simulink model "MicroMouseMatlab"  (R2024b)
settings: Solver=FixedStepAuto  StartTime=0.0  StopTime=0.1  RelTol=1e-3  EnableMultiTasking=on
undefined symbols (not defined in the file): samplingTime
settings Model: STM32="{\"DigitalPortWrite\":[{\"ID\":\"MicroMouseTemplate:84:3\"},{\"ID\":\"MicroMouseTemplate:84:4\"},{\"ID\":\"MicroMouseTemplate:84:5\"},{\"ID\":\"MicroMouseTemplate:84:6\"},{\"ID\":\"MicroMouseTemplate:84:7\"},{\"ID\":\"MicroMouseTemplate:84:8\"},{\"ID\":\"MicroMouseTemplate:84:9\"},{\"ID\":\"MicroMouseTemplate:84:10\"},{\"ID\":\"MicroMouseTemplate:160:19\"},{\"ID\":\"MicroMouseTemplate:2479:4\"},{\"ID\":\"MicroMouseTemplate:2479:6\"},{\"ID\":\"MicroMouseTemplate:2479:7\"},{\"ID\":\"MicroMouseTemplate:2479:8\"}],\"PWMOutput\":[{\"ID\":\"MicroMouseTemplate:160:24\"},{\"ID\":\"MicroMouseTemplate:160:25\"}],\"AnalogInput\":{\"ID\":\"MicroMouseTemplate:2357:1\"},\"DigitalPortRead\":[{\"ID\":\"MicroMouseTemplate:2483:3\"},{\"ID\":\"MicroMouseTemplate:2483:4\"}]}"  SimulationMode=external  ExtModeTrigDuration=10  Creator=JesseJabezArendse
settings SolverCC: AllowMultiTaskInputOutput=on  AutoInsertRateTranBlk=on  InsertRTBMode=Never (minimum delay)
settings OptimizationCC: EnhancedBackFolding=on  PassReuseOutputArgsAs=Individual arguments  StateBitsets=on  DataBitsets=on  ZeroExternalMemoryAtStartup=off  ZeroInternalMemoryAtStartup=off  NoFixptDivByZeroProtection=on  MaxStackSize=512  OptimizeBlockOrder=speed  DifferentSizesBufferReuse=on  EfficientTunableParamExpr=on
settings DebuggingCC: MultiTaskCondExecSysMsg=none  ParameterOverflowMsg=none  ParameterPrecisionLossMsg=none  ParameterTunabilityLossMsg=error
settings HardwareCC: ProdBitPerPointer=32  ProdBitPerSizeT=32  ProdBitPerPtrDiffT=32  ProdLargestAtomicInteger=Long  ProdLargestAtomicFloat=Double  ProdWordSize=32  ProdLongLongMode=on  ProdHWDeviceType=ARM Compatible->ARM Cortex  TargetBitPerLong=64  TargetBitPerPointer=64  TargetBitPerSizeT=64  TargetBitPerPtrDiffT=64  TargetLongLongMode=on  TargetIntDivRoundTo=Zero  TargetEndianess=LittleEndian  TargetWordSize=64  TargetHWDeviceType=MATLAB Host
settings ModelReferenceCC: EnableParallelModelReferenceBuilds=on  ParallelModelReferenceMATLABWorkerInit=Copy Base Workspace  SupportModelReferenceSimTargetCustomCode=on
settings SFSimCC: MATLABDynamicMemAlloc=off  SimHardwareAcceleration=native
settings RTWCC: Description=Embedded Coder  SystemTargetFile=ert.tlc  HardwareBoard=STM32L4xx Based  TLCOptions=-p0 -aInlineSetEventsForThisBaseRateFcn=TLC_FALSE -aSuppressMultiTaskScheduler=TLC_FALSE -aRateBasedStepFcn=1  TemplateMakefile=ert_default_tmf  Toolchain=GNU Tools for ARM Embedded Processors  CodeExecutionProfiling=on  CodeProfilingInstrumentation=coarse  GPUComputeCapability=3.5
settings RTWCC: CustomHeaderCode=|
  | #include "MicroMouseProgramming\Core\Inc\IMU.h"
  | #include "MicroMouseProgramming\Core\Inc\CustomWhile.h"
  | #include "MicroMouseProgramming\Core\Inc\Motors.h"
settings RTWCC: CustomInclude=|
  | MicroMouseProgramming\Core\Inc\
  | MicroMouseProgramming\Core\Src\
settings RTWCC: CustomSource=|
  | MicroMouseProgramming\Core\Src\IMU.c
  | MicroMouseProgramming\Core\Src\CustomWhile.c
  | MicroMouseProgramming\Core\Src\Motors.c
settings CodeAppCC: ForceParamTrailComments=on  IgnoreCustomStorageClasses=off  OperatorAnnotations=on  SimulinkDataObjDesc=on  SFDataObjDesc=on  InsertBlockDesc=on
settings ERTTargetCC: CodeReplacementLibrary=ARM Cortex-M  SupportNonFinite=off  SupportComplex=off  ExtModeTransport=3  ExtModeStaticAlloc=on  ExtModeStaticAllocSize=2048  ExtModeMexFile=ext_xcp  ExtModeIntrfLevel=Level2 - Open  InlinedParameterPlacement=Hierarchical  DynamicArrayContainerType=coder::array

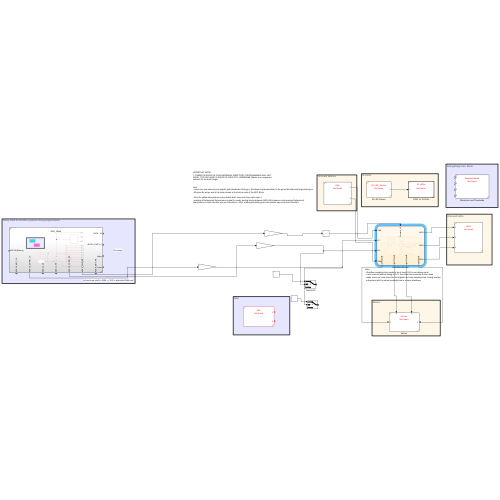
[thumbnail: Simulink's stored preview of the top-level diagram]
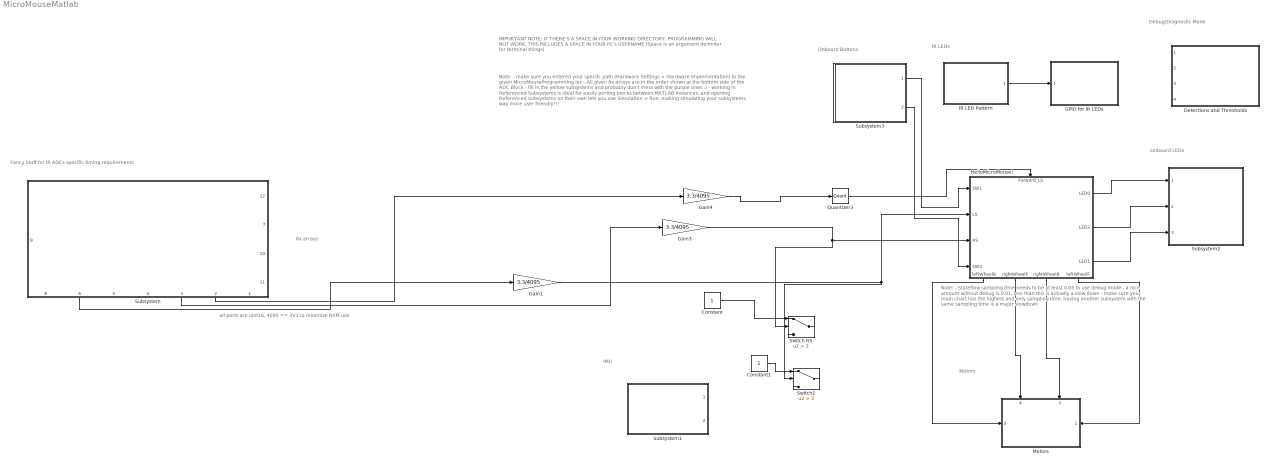
== system MicroMouseMatlab ==
  note: IMPORTANT NOTE:
      | IF THERE'S A SPACE IN YOUR WORKING DIRECTORY, PROGRAMMING WILL NOT WORK, THIS INCLUDES A SPACE IN YOUR PC's USERNAME (Space is an argument delimiter for terminal things)
  note: Note:
      | - make sure you entered your specifc path (Hardware Settings > Hardware Implementation) to the given MicroMouseProgramming.ioc
      | - All given 8x arrays are in the order shown at the bottom side of the ADC Block
      |
      | - fill in the yellow subsystems and probably don't mess with the purple ones :)
      | - working in Referenced Subsystems is ideal for easily porting blocks between MATLAB instances, and opening Referenced Subsystems on their own lets you use Simulation > Run, making simulating your subsystems way more user friendly!!!
  note: 8x arrays
  note: all ports are uint16, 4095 == 3V3 to minimize RAM use
  note: IMU
  note: Note:
      | - Stateflow sampling time needs to be at least 0.05 to use debug mode
      | - a nice amount without debug is 0.01, less than this is actually a slow down
      | - make sure your main chart has the highest and only sampling time, having another
      | subsystem with the same sampling time is a major slowdown
  note: Fancy Stuff for IR ADCs specific timing requirements
  note: IR LEDs
  note: Motors
  note: Onboard Buttons
  note: Onboard LEDs
  note: Debug/Diagnostic Mode
  Constant : Constant
  Constant1 : Constant
  Detections and Thresholds : Subsystem  ReferencedSubsystem=DiagnosticMode
  GPIO for IR LEDs : Subsystem  TreatAsAtomicUnit=on  SystemSampleTime=samplingTime  ReferencedSubsystem=IR_LEDs
  Gain1 : Gain  Gain=3.3/4095  OutDataTypeStr=single
  Gain3 : Gain  Gain=3.3/4095  OutDataTypeStr=single
  Gain4 : Gain  Gain=3.3/4095  OutDataTypeStr=single
  HelloMicroMouse! : Stateflow chart  TreatAsAtomicUnit=on
      settings: PortSchema="{\"entries\":[{\"content\":{\"sides\":[{\"content\":{\"connectorIds\":[\"In4\",\"In5\",\"In2\",\"In3\"]},\"type\":\"ConnectorPlacement.EquallySpacedRectSide\",\"uuid\":\"f52daa4f-6374-42e5-9ef1-0ccc99d09b58\"},{\"content\":{\"connectorIds\":[\"Out1\",\"Out2\",\"Out3\"],\"side\":\"RIGHT\"},\"type\":\"ConnectorPlacement.EquallySpacedRectSide\",\"uuid\":\"94b478cc-4dde-45c7-a588-77cf2b43cdb7\"},{\"content\":{\"connectorIds\":[\"In1\"],\"side\":\"TOP\"},\"type\":\"ConnectorPlacement.EquallySpacedRectSide\",\"uuid\":\"afff2079-ea5c-423e-9722-09c3bbce433b\"},{\"content\":{\"connectorIds\":[\"Out4\",\"Out5\",\"Out6\",\"Out7\"],\"side\":\"BOTTOM\"},\"type\":\"ConnectorPlacement.EquallySpacedRectSide\",\"uuid\":\"94e93a1d-795d-41a3-b2d8-d520b2bf47ef\"}]},\"type\":\"ConnectorPlacement.EquallySpacedConnector\",\"uuid\":\"d4d35636-54af-48ac-af70-d56caef5e090\"}],\"packageUris\":[\"http://schema.mathworks.com/mf0/Connector/R2020b\"],\"version\":\"1.0\"}"
  IR LED Pattern : Subsystem  ReferencedSubsystem=IR_LED_Pattern
  Motors : Subsystem  ReferencedSubsystem=Motors
      settings: PortSchema="{\"entries\":[{\"content\":{\"sides\":[{\"content\":{\"connectorIds\":[\"In2\"]},\"type\":\"ConnectorPlacement.EquallySpacedRectSide\",\"uuid\":\"bdd6fda3-7e00-416f-94f9-e16bb6cad3a7\"},{\"content\":{\"connectorIds\":[\"In1\"],\"side\":\"RIGHT\"},\"type\":\"ConnectorPlacement.EquallySpacedRectSide\",\"uuid\":\"976ec5aa-4295-418a-9a6a-f21268880cf4\"},{\"content\":{\"connectorIds\":[\"In4\",\"In3\"],\"side\":\"TOP\"},\"type\":\"ConnectorPlacement.EquallySpacedRectSide\",\"uuid\":\"6a8d0236-ba3b-4294-b9d1-b673d9586bad\"}]},\"type\":\"ConnectorPlacement.EquallySpacedConnector\",\"uuid\":\"379a3d58-51ae-4117-a8c6-ac947241712a\"}],\"packageUris\":[\"http://schema.mathworks.com/mf0/Connector/R2020b\"],\"version\":\"1.0\"}"
  Quantizer3 : Quantizer  QuantizationInterval=0.01
  Subsystem : Subsystem  ReferencedSubsystem=ADC_Block
      settings: PortSchema="{\"entries\":[{\"content\":{\"sides\":[{\"content\":{},\"type\":\"ConnectorPlacement.EquallySpacedRectSide\",\"uuid\":\"be6b81d5-7a49-4e34-b35f-0c07892094fc\"},{\"content\":{\"connectorIds\":[\"Out1\",\"Out2\",\"Out3\",\"Out4\",\"Out5\",\"Out6\",\"Out8\"],\"side\":\"RIGHT\"},\"type\":\"ConnectorPlacement.EquallySpacedRectSide\",\"uuid\":\"5e22590a-b7c0-4c63-8de4-8d81fd6c3849\"},{\"content\":{\"connectorIds\":[\"Out12\",\"Out7\",\"Out10\",\"Out11\"],\"side\":\"TOP\"},\"type\":\"ConnectorPlacement.EquallySpacedRectSide\",\"uuid\":\"da97636e-cea0-4a10-8fe5-d807f9ee999f\"},{\"content\":{\"connectorIds\":[\"Out9\"],\"side\":\"BOTTOM\"},\"type\":\"ConnectorPlacement.EquallySpacedRectSide\",\"uuid\":\"a593d780-81a8-4730-a8bc-2bbf356cafe4\"}]},\"type\":\"ConnectorPlacement.EquallySpacedConnector\",\"uuid\":\"0bcac921-e51a-4437-9183-315712d0a8c2\"}],\"packageUris\":[\"http://schema.mathworks.com/mf0/Connector/R2020b\"],\"version\":\"1.0\"}"
  Subsystem1 : Subsystem  ReferencedSubsystem=IMU
  Subsystem2 : Subsystem  ReferencedSubsystem=LEDs
  Subsystem3 : Subsystem  ReferencedSubsystem=SWs
  Switch RS : Switch  Criteria=u2 > Threshold  Threshold=3  SaturateOnIntegerOverflow=off  InputSameDT=off
  Switch1 : Switch  Criteria=u2 > Threshold  Threshold=3  SaturateOnIntegerOverflow=off  InputSameDT=off
  wires:
  Subsystem3/1 -> HelloMicroMouse!/4(SW1)
  Subsystem3/2 -> HelloMicroMouse!/3(SW2)
  IR LED Pattern/1 -> GPIO for IR LEDs/1
  HelloMicroMouse!/1(LED0) -> Subsystem2/1
  HelloMicroMouse!/5(rightWheelF) -> Motors/4
  Gain4/1 -> Quantizer3/1
  Quantizer3/1 -> HelloMicroMouse!/1(Forward_LS)
  Subsystem/2 -> Gain4/1
  Gain1/1 -> HelloMicroMouse!/5(LS), Switch1/2
  HelloMicroMouse!/4(leftWheelB) -> Motors/2
  HelloMicroMouse!/6(rightWheelB) -> Motors/3
  HelloMicroMouse!/7(leftWheelF) -> Motors/1
  Constant/1 -> Switch RS/1
  Gain3/1 -> Switch RS/2, HelloMicroMouse!/2(RS)
  Constant1/1 -> Switch1/1
  Subsystem/3 -> Gain3/1
  Subsystem/6 -> Gain1/1
  HelloMicroMouse!/2(LED2) -> Subsystem2/2
  HelloMicroMouse!/3(LED1) -> Subsystem2/3

== stateflow chart MicroMouseMatlab/HelloMicroMouse! ==
  state ButtonPressed
    state Move1
      entry:
      leftWheel = 3000;
      rightWheel = 3000;
      LED0 =false;
      LED1 =false;
      LED2 = false;
    state Calibration
      entry:
      Forward_LS = ADC14_FWD_LS;
      Right  = ADC11_RS;
      Left =  ADC12_LS;
      Forward_RS = ADC9_FWD_RS;
      Down_LS = ADC13_DOWN_LS;
      Down_RS = ADC10_DOWN_RS;
    state Stop
      entry:
      rightWheel = 0;
      leftWheel =0;
      LED0 =~ LED0;
      LED2 =~ LED2;
      LED1 =~ LED1;
    state Begin
      entry:
      LED0 =~ LED0;
      leftWheel = 0;
      rightWheel = 0;
    state LineFollow
      entry,during:
      if (Left >Right  )
      rightWheel = 3200;
      LeftWheel = 3000
      LED1 =true;
      end
      if (Left<Right )
      rightWheel = 3000;
      LeftWheel = 3200;
      LED2 = true;
      end
      if (Left>2.8 &&Right >2.8 && Forward_LS<ADC14_FWD_LS)
      rightWheel = 3000;
      LeftWheel =3000;
      LED1 =true;
      LED2 =true;
      end
    state Forward
      entry:
      LED0 = false
      LED2 = false;
      LED1 = false;
      rightWheel = 3000;
      leftWheel =3000;
    (default) -> (junction 77)
    (junction 77) -> Calibration [order 1] : [ (~ADC14_FWD_LS) && (~ADC11_RS) && (~ADC12_LS) ]
    (junction 77) -> (junction 79) [order 2]
    Move1 -> Stop : [after(0.7,sec)]
    Stop -> Move1 [order 2] : [Forward_LS >= ADC14_FWD_LS && Left >=ADC11_RS && Left >= ADC12_LS ]
    Calibration -> (junction 79)
    (junction 79) -> Begin
    (junction 130) -> Stop : [SW2]
    Begin -> (junction 130)
    (junction 132) -> Stop
    LineFollow -> (junction 132) [order 2] : [Forward_LS >ADC14_FWD_LS]
    Forward -> Stop [order 1] : [Forward_LS >ADC14_FWD_LS]
    Stop -> Forward [order 1] : [(Forward_LS < ADC14_FWD_LS && Right < ADC11_RS && Left < ADC12_LS) || (LS >= ADC12_LS && Right >= ADC11_RS && Forward_LS < ADC14_FWD_LS) ]
    Forward -> LineFollow [order 2] : [Left > Right  || Left <Right ]
    LineFollow -> Forward [order 1] : [after(0.2,sec)]
  state WaitUntilButtonPressed
    during:
  (default) -> WaitUntilButtonPressed
  WaitUntilButtonPressed -> ButtonPressed : [SW1]
  data: Forward_LS input; RS input; SW2 input; LED0 output; LED2 output; LED1 output; SW1 input; F local single; LS input; R local single; L local; leftWheelB output int16; rightWheelF output int16; rightWheelB output int16; leftWheelF output int16; ADC9_FWD_RS local; ADC14_FWD_LS local; ADC14_FWD_LS1 local
